simulink subsystem "Mode_Selector"  (R2025a)
settings: Solver=VariableStepAuto  StartTime=0.0  StopTime=10.0  RelTol=1e-3
undefined symbols (not defined in the file or in its folder): command, param1
libraries: px4uORBlib x3
settings Model: Creator=gurt1  LastModifiedBy=17036

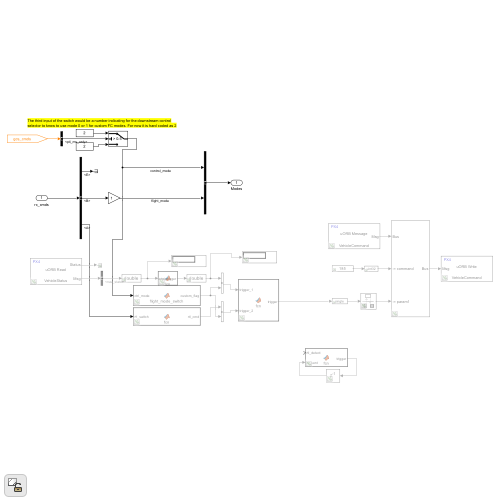
[thumbnail: Simulink's stored preview of the top-level diagram]
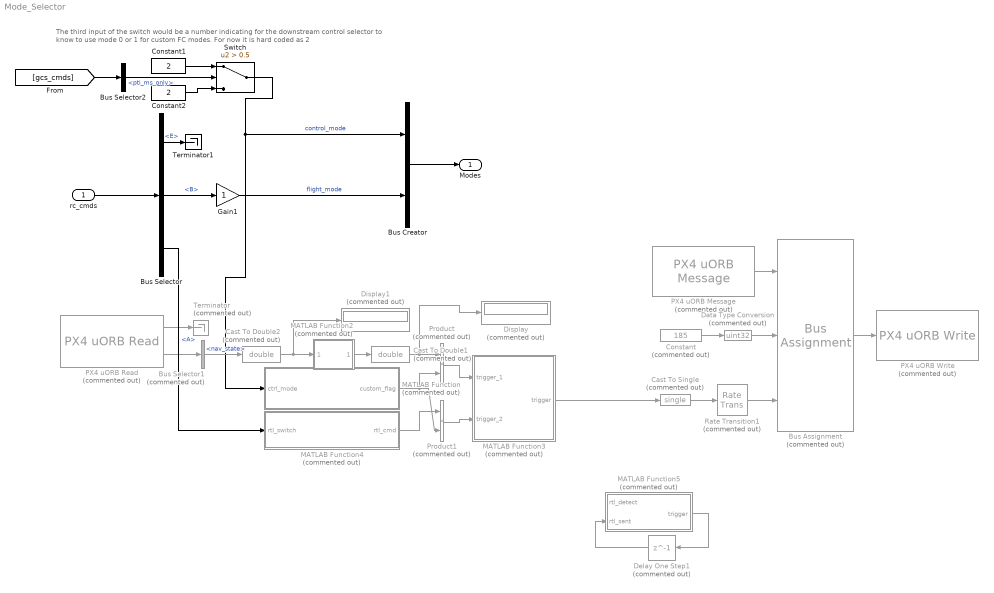
== system Mode_Selector ==
  note: The third input of the switch would be a number indicating for the downstream control selector to know to use mode 0 or 1 for custom FC modes. For now it is hard coded as 2
  rc_cmds : Inport
  Bus Assignment : BusAssignment  Commented=on  AssignedSignals=command,param1
  Bus Creator : BusCreator  Inputs=2
  Bus Selector : BusSelector  OutputSignals=switches.E,switches.B,switches.A
  Bus Selector1 : BusSelector  Commented=on  OutputSignals=nav_state
  Bus Selector2 : BusSelector  OutputSignals=PTI.PTI.ms.pti_ms_only
  Cast To Double1 : DataTypeConversion  Commented=on  OutDataTypeStr=double  SaturateOnIntegerOverflow=off  RndMeth=Floor
  Cast To Double2 : DataTypeConversion  Commented=on  OutDataTypeStr=double  SaturateOnIntegerOverflow=off  RndMeth=Floor
  Cast To Single : DataTypeConversion  Commented=on  OutDataTypeStr=single  SaturateOnIntegerOverflow=off  RndMeth=Floor
  Constant : Constant  Commented=on  Value=185
  Constant1 : Constant  Value=2
  Constant2 : Constant  Value=2
  Data Type Conversion : DataTypeConversion  Commented=on  OutDataTypeStr=uint32  SaturateOnIntegerOverflow=off  RndMeth=Floor
  Delay One Step1 : Delay  Commented=on  DelayLength=1
  Display : Display  Commented=on
  Display1 : Display  Commented=on
  Gain1 : Gain
  MATLAB Function : MATLAB Function  Commented=on  TreatAsAtomicUnit=on
  MATLAB Function2 : MATLAB Function  Commented=on  TreatAsAtomicUnit=on
  MATLAB Function3 : MATLAB Function  Commented=on  TreatAsAtomicUnit=on
  MATLAB Function4 : MATLAB Function  Commented=on  TreatAsAtomicUnit=on
  MATLAB Function5 : MATLAB Function  Commented=on  TreatAsAtomicUnit=on
  PX4 uORB Message : px4uORBlib/PX4 uORB Message  Commented=on  uORBTopic=VehicleCommand  SampleTime=1/4  selectInstance=vehicle_command
  PX4 uORB Read : px4uORBlib/PX4 uORB Read  Commented=on  uORBTopic=VehicleStatus  selectInstance=VehicleStatus  SampleTime=-1  BlockingMode=off  BlockTimeout=1e-3
  PX4 uORB Write : px4uORBlib/PX4 uORB Write  Commented=on  uORBTopic=VehicleCommand  selectInstance=vehicle_command  MessageQueueLen=1
  Product : Product  Commented=on
  Product1 : Product  Commented=on
  Rate Transition1 : RateTransition  Commented=on  OutPortSampleTime=1/4
  Switch : Switch  Criteria=u2 > Threshold  Threshold=0.5  SaturateOnIntegerOverflow=off  InputSameDT=off
  Terminator : Terminator  Commented=on
  Terminator1 : Terminator
  Modes : Outport
  wires:
  rc_cmds/1 -> Bus Selector/1
  Bus Creator/1 -> Modes/1
  Bus Selector/1 -> Terminator1/1  "<E>"
  Bus Selector/2 -> Gain1/1  "<B>"
  Switch/1 -> Bus Creator/1, MATLAB Function/1(ctrl_mode)  "control_mode"
  Gain1/1 -> Bus Creator/2  "flight_mode"
  PX4 uORB Read/1 -> Terminator/1
  PX4 uORB Read/2 -> Bus Selector1/1
  Bus Selector1/1 -> Cast To Double2/1  "<nav_state>"
  Cast To Double2/1 -> Display1/1, MATLAB Function2/1(state)
  MATLAB Function2/1(term_trigger) -> Cast To Double1/1
  Cast To Double1/1 -> Product/1, Display/1
  MATLAB Function/1(custom_flag) -> Product/2, Product1/2
  PX4 uORB Message/1 -> Bus Assignment/1
  Constant/1 -> Data Type Conversion/1
  Data Type Conversion/1 -> Bus Assignment/2
  Cast To Single/1 -> Rate Transition1/1
  Bus Assignment/1 -> PX4 uORB Write/1
  Rate Transition1/1 -> Bus Assignment/3
  MATLAB Function3/1(trigger) -> Cast To Single/1
  Product/1 -> MATLAB Function3/1(trigger_1)
  Bus Selector/3 -> MATLAB Function4/1(rtl_switch)  "<A>"
  MATLAB Function5/1(trigger) -> Delay One Step1/1
  Delay One Step1/1 -> MATLAB Function5/2(rtl_sent)
  Product1/1 -> MATLAB Function3/2(trigger_2)
  MATLAB Function4/1(rtl_cmd) -> Product1/1
  [gcs_cmds] -> Bus Selector2/1
  Bus Selector2/1 -> Switch/2  "<pti_ms_only>"
  Constant1/1 -> Switch/1
  Constant2/1 -> Switch/3

== matlab function Mode_Selector/MATLAB Function2 ==
  data: state input; term_trigger output
function term_trigger = fcn(state)

if state == 18 || state == 5 || state == 13
    term_trigger = 1;
else 
    term_trigger = 0;
end

== matlab function Mode_Selector/MATLAB Function3 ==
  data: trigger_1 input; trigger output; trigger_2 input
function trigger = fcn(trigger_1,trigger_2)

if trigger_1 >= 0.5 || trigger_2 >= 0.5
    trigger = 1;
else 
    trigger = 0;
end

== matlab function Mode_Selector/MATLAB Function4 ==
  data: rtl_switch input; rtl_cmd output
function rtl_cmd = fcn(rtl_switch)

if rtl_switch >= 0.5
    rtl_cmd = 1;
else
    rtl_cmd = 0;
end

== matlab function Mode_Selector/MATLAB Function5 ==
  data: trigger output; rtl_detect input; rtl_sent input
function trigger = fcn(rtl_detect,rtl_sent)

if rtl_detect >= 0.5 && rtl_sent <= 0.5
    trigger = 1;
elseif rtl_detect >= 0.5 && rtl_sent >= 0.5
    trigger = 0;
else
    trigger = 0;
end

== matlab function Mode_Selector/MATLAB Function ==
  data: ctrl_mode input; custom_flag output
function custom_flag = flight_mode_switch(ctrl_mode)
    if ctrl_mode >= 0.5
        custom_flag = 0;
    else
        custom_flag = 1;
    end
end
